simulink model "unload_load_protocol"  (R2022a)
settings: Solver=VariableStepAuto  StartTime=0.0  StopTime=10.0  RelTol=1e-3
settings Model: NumberOfSteps=10  Creator=rodri  LastModifiedBy=rodri

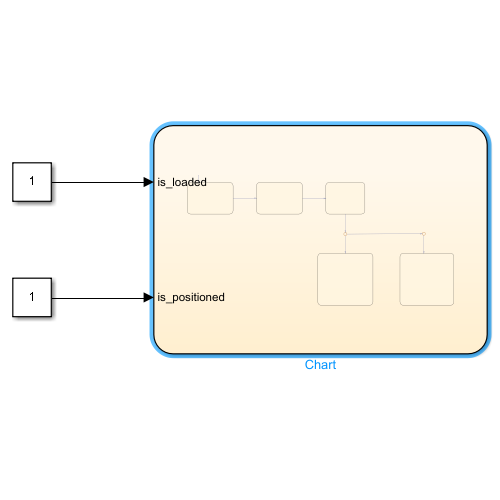
[thumbnail: Simulink's stored preview of the top-level diagram]
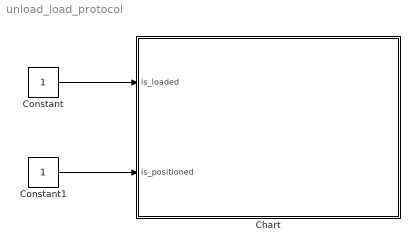
== system unload_load_protocol ==
  Chart : Stateflow chart  TreatAsAtomicUnit=on
  Constant : Constant
  Constant1 : Constant
  wires:
  Constant/1 -> Chart/1(is_loaded)
  Constant1/1 -> Chart/2(is_positioned)

== stateflow chart unload_load_protocol/Chart ==
  note: Lado é determinado pela Ordem de Serviço
  state Delivering
  state ApproachingTables
    entry:
    set_speed_loading();
    rise_curtains();
  state AligningToTables
    entry:
    set_speed_aligning();
    shut_down_ultrasounds();
  state Unloading
    note: %Flag apenas para lever alto
    state MotorsOff
    state MotorOn
      entry:
      motor_on(unload);
    (default) -> Unloading.MotorsOff : {set_bars(-1);
        | send_cmd_table_motors_on();}
    Unloading.MotorsOff -> Unloading.MotorOn [order 1] : [get_table_motors_state() & ...
        | is_bars_down()]
    Unloading.MotorOn -> Unloading.MotorsOff : [is_table_loaded]
  state Loading
    state MotorsOff
    state MotorOn
      entry:
      send_cmd_table_motors_on()
    (default) -> Loading.MotorsOff : {set_bars(-1);}
    Loading.MotorsOff -> Loading.MotorOn : [is_bars_down()]{motor_on(load);}
    Loading.MotorOn -> Loading.MotorsOff [order 2] : [~get_table_motors_state()]{warning_table_motors()}
  (default) -> Delivering
  Delivering -> ApproachingTables : [check_location]
  ApproachingTables -> AligningToTables : [is_positioned]
  AligningToTables -> (junction 7) : [vehicle_positioned()]
      | {stop_vehicle()}
  (junction 45) -> Delivering
  (junction 7) -> (junction 11) [order 2]
  (junction 11) -> Loading
  (junction 7) -> Unloading [order 1] : [is_loaded]
  Unloading.MotorsOff -> (junction 32) [order 2] : [is_vehicle_clear]
      | {set_bars(1);}
  Loading.MotorOn -> (junction 36) [order 1] : [get_table_motors_state() & is_vehicle_loaded]
      | {raise_bars();}
  (junction 32) -> (junction 45) : [is_payload_safe()]
  (junction 36) -> (junction 32)
  data: is_loaded input; is_positioned input; check_location local =1
  function set_speed_loading:
    | function set_speed_loading()
    | % Externo ao galpao deve ser de 50m/min = 83 cm/s
    | % Dentro do galpao deve ser de 30m/min = 50 cm/s
    | % Aproximando da mesa deve ser de 20m/min
    | % Ajuste fino na mesa deve ser em 3m/min
    | 
    |     speed_now = 90 * 0.5;
    |     disp("Speed now is " + string(speed_now))
    | end
  function rise_curtains:
    | function rise_curtains
    | 
    | disp("Rising Curtains")
    | pause(2);
    | disp("Curtains rised")
